simulink model "IngenuityExperiment"  (R2023a)
settings: Solver=VariableStepAuto  StartTime=0.0  StopTime=0.3  RelTol=1e-3
libraries: simulink x1, aerolibpropulsion2 x1
settings Model: Creator=vboutrou  LastModifiedBy=vboutrou

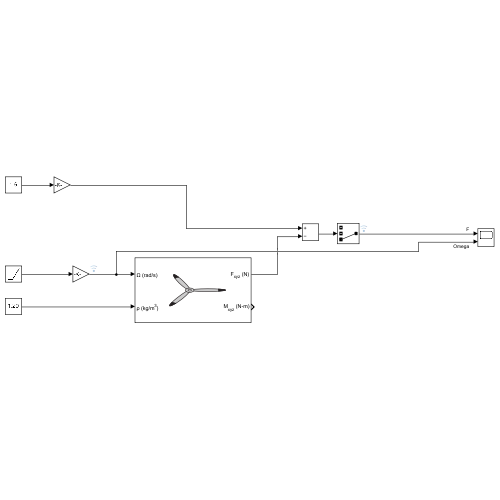
[thumbnail: Simulink's stored preview of the top-level diagram]
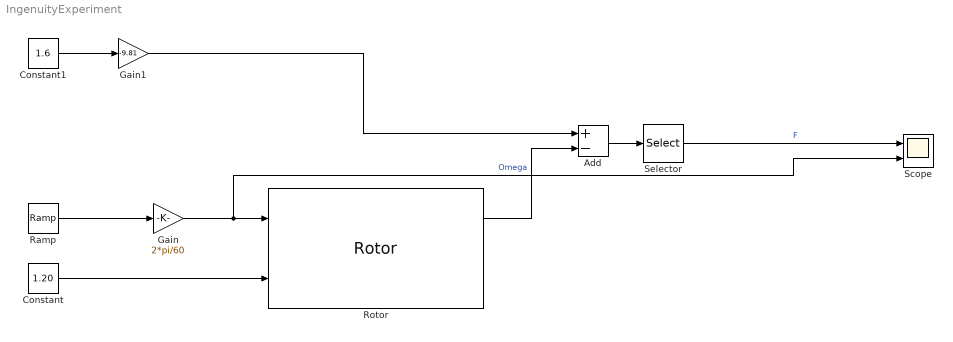
== system IngenuityExperiment ==
  Add : Sum  Inputs=+-
  Constant : Constant  Value=1.20
  Constant1 : Constant  Value=1.6
  Gain : Gain  Gain=2*pi/60
  Gain1 : Gain  Gain=-9.81
  Ramp : simulink/Sources/Ramp  slope=1000  start=0  InitialOutput=0
  Rotor : aerolibpropulsion2/Rotor  units=Metric (MKS)  modelMode=Without flap effects  blockSelect=Single  config=Quadcopter X  Nr=1  l=0.0624  h=-0.0159  Arm=[0;0;0]  Nb=2  CTcheck=off  CT=0.0175  CQ=7.8263e-4  CTout=off  R=1.0  c=0.0080  e=0  clalpha=5.5  gamma=0.6051  twistType=Linear  theta0=0.2548  theta1=-0.1361  thetaTip=0.1018  Vb=[0;0;0]  pqr=[0;0;0]
      settings: LibrarySourceBlock=aerolibrotor/Rotor
  Scope : Scope  NumInputPorts=2
  Selector : Selector  InputPortWidth=3  IndexOptions=Index vector (dialog)  Indices=[3]  OutputSizes=1
  wires:
  Ramp/1 -> Gain/1
  Gain/1 -> Scope/2, Rotor/1  "Omega"
  Constant/1 -> Rotor/2
  Constant1/1 -> Gain1/1
  Gain1/1 -> Add/1
  Rotor/1 -> Add/2
  Add/1 -> Selector/1
  Selector/1 -> Scope/1  "F"
